simulink model "LED_TX"  (R2017b)
settings: Solver=VariableStepAuto  StartTime=0.0  StopTime=8099  RelTol=1e-3
undefined symbols (not defined in the file or in its folder): get, hot
libraries: visionsources x3, simulink x3, SimulinkLED1v4 x3, dspsnks4 x1
settings Model: Creator=asus  LastModifiedBy=asus

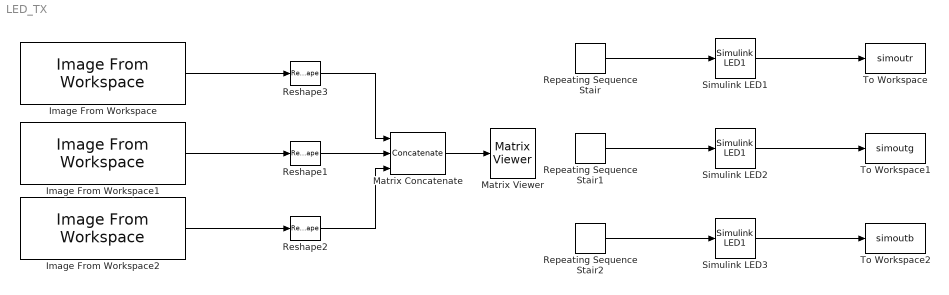
== system LED_TX ==
  Image From Workspace : visionsources/Image From Workspace  Tag=vipblks_nd  ImageValue=simoutr  Ts=1  imagePorts=One multidimensional signal  OutPortLabels=R  ImageDataType=Inherit from 'Value'  Signed=on  WordLength=16  sdImageDataType=sfix(16)  FractionLengthMode=User-defined  FractionLength=15
      settings: SourceProductName=Computer Vision System Toolbox  SourceProductBaseCode=VP
  Image From Workspace1 : visionsources/Image From Workspace  Tag=vipblks_nd  ImageValue=simoutg  Ts=1  imagePorts=One multidimensional signal  OutPortLabels=G  ImageDataType=Inherit from 'Value'  Signed=on  WordLength=16  sdImageDataType=sfix(16)  FractionLengthMode=User-defined  FractionLength=15
      settings: SourceProductName=Computer Vision System Toolbox  SourceProductBaseCode=VP
  Image From Workspace2 : visionsources/Image From Workspace  Tag=vipblks_nd  ImageValue=simoutb  Ts=1  imagePorts=One multidimensional signal  OutPortLabels=B  ImageDataType=Inherit from 'Value'  Signed=on  WordLength=16  sdImageDataType=sfix(16)  FractionLengthMode=User-defined  FractionLength=15
      settings: SourceProductName=Computer Vision System Toolbox  SourceProductBaseCode=VP
  Matrix Concatenate : Concatenate  NumInputs=3  Mode=Multidimensional array  ConcatenateDimension=2
  Matrix Viewer : dspsnks4/Matrix Viewer  ImageParams=off  CMapStr=hot(256)  AxisColorbar=off  AxisParams=off  AxisOrigin=Upper left corner  AxisTickMode=Auto  XTickRange=[0 1]  YTickRange=[0 1]  XLabel=RGB colors  YLabel=Pixel values  ZLabel=Z-axis  FigPos=get(0,'defaultfigureposition')  AxisZoom=off
      settings: SourceProductName=DSP System Toolbox  SourceProductBaseCode=DS  YMin=0  YMax=255
  Repeating Sequence Stair : simulink/Sources/Repeating Sequence Stair  OutValues=[251,107,54,59,59,59,59,59,59,59,59,59,59,59,59,59,59,59,59,59,59,59,59,59,59,59,59,59,59,59,59,59,59,59,59,59,59,59,59,59,59,59,54,107,255,198,56,59,59,59,59,59,59,59,59,59,59,59,59,59,59,59,59,59,59,59,59,59,59,59,59,59,59,59,59,59,59,59,59,59,59,59,59,59,59,59,59,59,56,204,156,51,59,59,59,59,59,59,59,59,59,59,59,59,59,59,59,59,59,59,59,58,58,58,58,59,59,59,59,59,59,59,59,59,59,59,59,59,59,59,59,59,59,51,154,125,53,59,59,59,59,59,59,59,59,59,59,59,59,59,59,59,59,59,58,58,58,58,58,58,58,58,59,59,59,59,59,59,59,59,59,59,59,59,59,59,59,59,54,113,99,55,59,59,59,59,59,59,59,59,59,59,59,59,59,59,59,59,58,58,58,58,58,58,58,58,58,58,59,59,59,59,59,59,59,59,59,59,59,59,59,59,59,56,85,82,57,59,59,59,59,59,59,59,59,59,59,59,59,59,59,59,58,58,58,58,58,58,58,58,58,58,58,58,59,59,59,59,59,59,59,59,59,59,59,59,59,59,58,70,69,58,59,59,59,59,59,59,59,59,59,59,59,59,59,59,58,58,58,58,58,58,57,57,58,58,58,58,58,58,59,59,59,59,59,59,59,59,59,59,59,59,59,59,60,60,59,59,59,59,59,59,59,59,59,59,59,59,59,59,59,58,58,58,58,57,57,57,57,57,57,58,58,58,58,58,59,59,59,59,59,59,59,59,59,59,59,59,59,59,59,59,59,59,59,59,59,59,59,59,59,59,59,59,59,58,58,58,58,57,57,57,57,57,57,57,57,57,58,58,58,59,59,59,59,59,59,59,59,59,59,59,59,59,59,59,59,59,59,59,59,59,59,59,59,59,59,59,59,58,58,58,58,57,57,57,57,57,57,57,57,57,57,57,58,58,58,59,59,59,59,59,59,59,59,59,59,59,59,59,59,59,59,59,59,59,59,59,59,59,59,59,59,59,58,58,58,57,57,57,56,56,56,56,56,56,57,57,57,57,58,58,58,59,59,59,59,59,59,59,59,59,59,59,59,59,59,59,59,59,59,59,59,59,59,59,59,59,58,58,58,57,57,57,56,56,56,56,56,56,56,56,56,57,57,58,58,58,59,59,59,59,59,59,59,59,59,59,59,59,59,59,59,59,59,59,59,59,59,59,59,59,59,58,58,58,57,57,56,56,56,56,56,56,56,56,56,56,56,57,57,58,58,58,59,59,59,59,59,59,59,59,59,59,59,59,59,59,59,59,59,59,59,59,59,59,59,58,58,58,57,57,56,56,56,55,55,55,55,55,55,56,56,56,57,57,57,58,58,59,59,59,59,59,59,59,59,59,59,59,59,59,59,59,59,59,59,59,59,59,59,59,58,58,57,57,56,56,56,55,55,55,55,55,55,55,55,56,56,56,57,57,58,58,58,59,59,59,59,59,59,59,59,59,59,59,59,59,59,59,59,59,59,59,59,59,59,58,58,57,56,56,56,55,55,55,54,54,54,54,54,55,55,56,56,56,57,57,58,58,59,59,59,59,59,59,59,59,59,59,59,59,59,59,59,59,59,59,59,59,59,58,58,57,57,56,56,55,55,54,54,54,54,54,54,54,54,55,55,56,56,56,57,58,58,59,59,59,59,59,59,59,59,59,59,59,59,59,59,59,59,59,59,59,59,59,58,58,57,56,56,55,55,54,54,54,54,53,53,53,54,54,54,55,55,56,56,57,57,58,58,59,59,59,59,59,59,59,59,59,59,59,59,59,59,59,59,59,59,59,58,58,57,57,56,56,55,54,54,54,53,53,53,53,53,53,53,54,54,55,55,56,56,57,58,58,59,59,59,59,59,59,59,59,59,59,59,59,59,59,59,59,59,59,59,58,58,57,56,56,55,55,54,54,52,60,103,122,104,60,52,53,53,54,54,55,56,56,57,58,58,59,59,59,59,59,59,59,59,59,59,59,59,59,59,59,59,59,59,59,58,58,57,56,56,55,54,53,52,121,208,221,219,220,209,122,53,53,53,54,54,55,56,57,57,58,58,59,59,59,59,59,59,59,59,59,59,59,59,59,59,59,59,59,58,58,57,57,56,55,54,53,55,154,222,219,219,220,220,220,224,156,55,52,53,54,55,56,56,57,58,58,59,59,59,59,59,59,59,59,59,59,59,59,59,59,59,59,59,58,58,57,56,56,55,54,51,150,223,219,219,220,220,220,220,220,225,151,51,53,54,54,55,56,56,57,58,59,59,59,59,59,59,59,59,59,59,59,59,59,59,59,59,59,58,58,57,56,55,54,49,118,221,219,220,220,220,221,221,221,221,221,222,119,48,53,54,55,56,56,57,58,58,59,59,59,59,59,59,59,59,59,59,59,59,59,59,59,58,58,57,56,56,55,51,76,205,221,219,220,220,221,221,221,221,221,221,223,208,77,50,54,54,55,56,57,58,58,59,59,59,59,59,59,59,59,59,59,59,59,59,59,59,58,58,57,56,55,54,51,161,224,219,220,221,221,222,222,222,222,222,222,221,226,163,51,53,54,55,56,57,57,58,59,59,59,59,59,59,59,59,59,59,59,59,59,59,59,58,58,56,56,55,50,95,217,220,220,220,221,222,222,222,223,223,222,222,222,222,220,96,48,54,54,56,56,57,58,58,59,59,59,59,59,59,59,59,59,59,59,59,59,59,58,57,56,56,54,52,169,224,219,220,221,222,222,223,223,223,223,223,223,222,222,226,172,52,53,54,55,56,57,58,58,59,59,59,59,59,59,59,59,59,59,59,59,59,58,58,57,56,55,50,92,217,220,220,221,222,222,223,223,223,224,224,224,223,223,223,223 ...(+23997 chars)]  tsamp=1  OutMin=[]  OutMax=[]  OutDataTypeStr=double  OutputDataTypeScalingMode=double  OutDataType=fixdt(0,8)  ConRadixGroup=Best Precision: Vector-wise  OutScaling=2^-12
  Repeating Sequence Stair1 : simulink/Sources/Repeating Sequence Stair  OutValues=[251,130,85,89,89,89,89,89,89,89,89,89,89,89,89,89,89,89,89,89,89,89,88,88,89,89,89,89,89,89,89,89,89,89,89,89,89,89,89,89,89,89,85,130,255,207,86,89,89,89,89,89,89,89,89,89,89,89,89,89,89,89,89,89,89,88,88,88,88,88,88,88,89,89,89,89,89,89,89,89,89,89,89,89,89,89,89,89,87,212,171,82,89,89,89,89,89,89,89,89,89,89,89,89,89,89,89,89,89,88,88,88,88,88,88,88,88,88,89,89,89,89,89,89,89,89,89,89,89,89,89,89,89,83,170,145,84,89,89,89,89,89,89,89,89,89,89,89,89,89,89,89,89,88,88,88,88,88,88,88,88,88,88,88,89,89,89,89,89,89,89,89,89,89,89,89,89,89,85,135,123,85,89,89,89,89,89,89,89,89,89,89,89,89,89,89,89,88,88,88,88,88,87,87,88,88,88,88,88,88,89,89,89,89,89,89,89,89,89,89,89,89,89,87,111,108,87,89,89,89,89,89,89,89,89,89,89,89,89,89,89,88,88,88,88,87,87,87,87,87,87,88,88,88,88,88,89,89,89,89,89,89,89,89,89,89,89,89,88,99,97,88,89,89,89,89,89,89,89,89,89,89,89,89,89,88,88,88,88,87,87,87,87,87,87,87,87,87,88,88,88,89,89,89,89,89,89,89,89,89,89,89,89,89,90,90,89,89,89,89,89,89,89,89,89,89,89,89,89,88,88,88,88,87,87,87,87,86,86,86,87,87,87,87,88,88,88,89,89,89,89,89,89,89,89,89,89,89,89,89,89,89,89,89,89,89,89,89,89,89,89,89,89,89,88,88,88,87,87,87,86,86,86,86,86,86,86,87,87,87,88,88,88,89,89,89,89,89,89,89,89,89,89,89,89,89,89,89,89,89,89,89,89,89,89,89,89,89,88,88,88,87,87,87,86,86,86,86,86,86,86,86,86,87,87,88,88,88,89,89,89,89,89,89,89,89,89,89,89,89,89,89,89,89,89,89,89,89,89,89,89,89,89,88,88,87,87,87,86,86,85,85,85,85,85,85,86,86,86,87,87,88,88,88,89,89,89,89,89,89,89,89,89,89,89,89,89,89,89,89,89,89,89,89,89,89,89,88,88,88,87,87,86,86,85,85,85,84,84,85,85,85,85,86,86,87,87,88,88,89,89,89,89,89,89,89,89,89,89,89,89,89,89,89,89,89,89,89,89,89,89,89,88,88,87,87,86,86,85,85,84,84,84,84,84,84,85,85,85,86,87,87,88,88,88,89,89,89,89,89,89,89,89,89,89,89,89,89,89,89,89,89,89,89,89,89,88,88,88,87,86,86,85,85,84,83,83,83,83,83,83,84,84,85,86,86,87,87,88,88,89,89,89,89,89,89,89,89,89,89,89,89,89,89,89,89,89,89,89,89,89,88,88,87,87,86,85,85,84,83,83,83,82,82,82,83,83,83,84,85,86,86,87,88,88,89,89,89,89,89,89,89,89,89,89,89,89,89,89,89,89,89,89,89,89,89,88,88,87,86,85,85,84,83,83,82,82,82,82,82,82,83,83,83,85,85,86,87,87,88,88,89,89,89,89,89,89,89,89,89,89,89,89,89,89,89,89,89,89,89,88,88,87,87,86,85,84,83,83,82,82,81,81,81,81,82,82,82,83,83,85,86,86,87,88,88,89,89,89,89,89,89,89,89,89,89,89,89,89,89,89,89,89,89,89,88,88,87,86,85,84,83,83,82,81,81,81,81,81,81,81,81,82,82,83,84,85,86,87,87,88,88,89,89,89,89,89,89,89,89,89,89,89,89,89,89,89,89,89,89,88,87,87,86,85,84,83,82,81,81,81,80,80,80,80,80,81,81,82,82,83,84,85,86,87,88,88,89,89,89,89,89,89,89,89,89,89,89,89,89,89,89,89,89,88,88,87,86,85,84,83,82,81,81,79,86,122,138,122,86,79,80,81,81,82,83,84,85,86,87,88,88,89,89,89,89,89,89,89,89,89,89,89,89,89,89,89,89,89,88,88,87,86,85,84,82,82,81,80,137,210,220,219,220,210,137,80,80,81,81,82,83,84,85,87,87,88,88,89,89,89,89,89,89,89,89,89,89,89,89,89,89,89,89,88,87,87,86,84,83,82,80,82,165,222,219,219,220,220,220,223,166,82,79,81,81,82,84,85,86,87,88,88,89,89,89,89,89,89,89,89,89,89,89,89,89,89,89,88,88,87,86,85,84,82,81,79,161,222,219,219,220,220,220,220,220,224,162,78,80,81,82,83,84,86,87,88,88,89,89,89,89,89,89,89,89,89,89,89,89,89,89,89,88,88,87,86,84,83,82,77,134,220,219,220,220,220,221,221,221,221,221,222,135,76,80,82,82,84,85,86,87,88,88,89,89,89,89,89,89,89,89,89,89,89,89,89,89,88,87,86,85,84,82,79,99,207,220,219,220,220,221,221,221,221,221,221,222,210,99,77,81,82,83,85,86,87,88,88,89,89,89,89,89,89,89,89,89,89,89,89,89,88,88,87,86,85,83,82,79,171,223,219,220,221,221,222,222,222,222,222,222,221,225,172,78,80,81,82,84,86,87,88,88,89,89,89,89,89,89,89,89,89,89,89,89,89,88,88,87,86,84,83,78,115,217,220,220,220,221,222,222,222,223,223,222,222,222,222,220,115,76,81,82,84,85,86,87,88,89,89,89,89,89,89,89,89,89,89,89,89,89,88,88,86,85,84,82,80,177,223,219,220,221,222,222,223,223,223,223,223,223,222,222,226,179,78,80,82,83,84,86,87,88,88,89,89,89,89,89,89,89,89,89,89,89,89,88,87,86,85,83,78,113,217,220,220,221,222,222,223,223,223,224,224,224,223,223 ...(+24118 chars)]  tsamp=1  OutMin=[]  OutMax=[]  OutDataTypeStr=double  OutputDataTypeScalingMode=double  OutDataType=fixdt(0,8)  ConRadixGroup=Best Precision: Vector-wise  OutScaling=2^-12
  Repeating Sequence Stair2 : simulink/Sources/Repeating Sequence Stair  OutValues=[253,177,150,152,152,152,152,152,152,152,152,152,152,152,152,152,152,152,151,151,151,151,151,151,151,151,151,151,151,152,152,152,152,152,152,152,152,152,152,152,152,152,150,177,255,225,150,152,152,152,152,152,152,152,152,152,152,152,152,152,152,152,151,151,151,151,151,151,151,151,151,151,151,151,151,152,152,152,152,152,152,152,152,152,152,152,152,152,150,228,203,148,152,152,152,152,152,152,152,152,152,152,152,152,152,152,151,151,151,151,151,150,150,150,150,151,151,151,151,151,151,152,152,152,152,152,152,152,152,152,152,152,152,148,202,187,149,152,152,152,152,152,152,152,152,152,152,152,152,152,151,151,151,151,150,150,150,150,150,150,150,150,151,151,151,151,152,152,152,152,152,152,152,152,152,152,152,152,149,180,173,150,152,152,152,152,152,152,152,152,152,152,152,152,151,151,151,151,150,150,150,150,149,149,150,150,150,150,151,151,151,151,152,152,152,152,152,152,152,152,152,152,152,151,166,164,151,152,152,152,152,152,152,152,152,152,152,152,152,151,151,151,150,150,150,149,149,148,148,149,149,150,150,150,151,151,151,151,152,152,152,152,152,152,152,152,152,152,151,158,157,151,152,152,152,152,152,152,152,152,152,152,152,151,151,151,150,150,150,149,148,148,148,148,148,148,148,149,150,150,151,151,151,152,152,152,152,152,152,152,152,152,152,152,153,152,152,152,152,152,152,152,152,152,152,152,152,152,151,151,151,150,150,149,148,148,148,147,147,147,148,148,148,149,150,150,151,151,151,152,152,152,152,152,152,152,152,152,152,152,152,152,152,152,152,152,152,152,152,152,152,152,151,151,151,150,150,149,148,148,147,147,147,147,147,147,147,148,148,149,150,151,151,151,152,152,152,152,152,152,152,152,152,152,152,152,152,152,152,152,152,152,152,152,152,152,152,151,151,150,150,149,148,147,147,147,146,146,146,146,146,147,147,148,148,150,150,151,151,151,152,152,152,152,152,152,152,152,152,152,152,152,152,152,152,152,152,152,152,152,152,151,151,151,150,149,148,147,147,146,145,145,145,145,145,145,145,147,147,148,148,150,150,151,151,152,152,152,152,152,152,152,152,152,152,152,152,152,152,152,152,152,152,152,152,152,151,151,150,150,148,148,147,146,145,145,144,144,144,144,144,145,145,146,147,148,149,150,151,151,151,152,152,152,152,152,152,152,152,152,152,152,152,152,152,152,152,152,152,152,151,151,151,150,149,148,147,146,145,144,144,143,143,143,143,143,144,145,145,147,148,148,150,150,151,151,152,152,152,152,152,152,152,152,152,152,152,152,152,152,152,152,152,152,152,151,151,150,149,148,147,146,145,144,143,143,143,142,142,142,143,143,144,144,146,147,148,149,150,151,151,151,152,152,152,152,152,152,152,152,152,152,152,152,152,152,152,152,152,152,151,151,150,149,148,147,145,144,143,143,141,141,141,141,141,141,142,143,144,145,146,147,148,149,150,151,151,152,152,152,152,152,152,152,152,152,152,152,152,152,152,152,152,152,151,151,151,150,148,147,146,144,144,142,141,141,140,140,140,140,140,141,142,143,144,145,146,148,149,150,151,151,152,152,152,152,152,152,152,152,152,152,152,152,152,152,152,152,152,151,151,150,149,148,146,145,144,142,141,140,140,139,139,139,139,139,140,141,142,143,144,146,147,148,150,151,151,151,152,152,152,152,152,152,152,152,152,152,152,152,152,152,152,152,151,151,150,148,147,145,144,143,141,140,139,138,138,138,138,138,138,139,140,141,142,144,144,146,148,149,150,151,151,152,152,152,152,152,152,152,152,152,152,152,152,152,152,152,151,151,150,149,148,146,144,143,142,141,139,138,138,137,137,137,137,137,138,139,140,141,142,144,145,147,148,150,151,151,152,152,152,152,152,152,152,152,152,152,152,152,152,152,152,151,151,150,149,147,145,144,142,141,139,138,137,141,161,170,161,140,136,137,138,139,140,141,143,144,146,148,149,151,151,151,152,152,152,152,152,152,152,152,152,152,152,152,152,152,151,151,149,148,146,145,143,141,140,138,137,170,213,220,219,220,214,170,136,137,138,139,140,142,144,145,147,149,150,151,151,152,152,152,152,152,152,152,152,152,152,152,152,152,151,151,150,149,148,146,144,142,140,138,138,187,220,219,219,220,220,220,222,187,137,137,138,139,141,143,145,147,148,150,151,151,152,152,152,152,152,152,152,152,152,152,152,152,152,151,151 ...(+28404 chars)]  tsamp=1  OutMin=[]  OutMax=[]  OutDataTypeStr=double  OutputDataTypeScalingMode=double  OutDataType=fixdt(0,8)  ConRadixGroup=Best Precision: Vector-wise  OutScaling=2^-12
  Reshape1 : Reshape  OutputDimensionality=Customize  OutputDimensions=[90,90]
  Reshape2 : Reshape  OutputDimensionality=Customize  OutputDimensions=[90,90]
  Reshape3 : Reshape  OutputDimensionality=Customize  OutputDimensions=[90,90]
  Simulink LED1 : SimulinkLED1v4/Simulink LED1  Description=|  outportflag=on  IconShape=Triangle  range1=[0 255]  color1=Red  range2=[100 255]  color2=Green  colorRest=Blue
      | -ranges-
      | (-inf 0]
      settings: AttributesFormatString=%<Description>  SourceProductName=The database C:\Users\asus\AppData\Roaming\MathWorks\MATLAB\R2017b\slblocks_master.db is locked, or a table in the database is locked. (database is locked)
  Simulink LED2 : SimulinkLED1v4/Simulink LED1  Description=|  outportflag=on  IconShape=Triangle  range1=[0 255]  color1=Red  range2=[100 255]  color2=Green  colorRest=Blue
      | -ranges-
      | (-inf 0]
      settings: AttributesFormatString=%<Description>  SourceProductName=The database C:\Users\asus\AppData\Roaming\MathWorks\MATLAB\R2017b\slblocks_master.db is locked, or a table in the database is locked. (database is locked)
  Simulink LED3 : SimulinkLED1v4/Simulink LED1  Description=|  outportflag=on  IconShape=Triangle  range1=[0 255]  color1=Red  range2=[100 255]  color2=Green  colorRest=Blue
      | -ranges-
      | (-inf 0]
      settings: AttributesFormatString=%<Description>  SourceProductName=The database C:\Users\asus\AppData\Roaming\MathWorks\MATLAB\R2017b\slblocks_master.db is locked, or a table in the database is locked. (database is locked)
  To Workspace : ToWorkspace  VariableName=simoutr  SampleTime=1
      settings: Save2DSignal=2-D array (concatenate along first dimension)
  To Workspace1 : ToWorkspace  VariableName=simoutg  SampleTime=1
      settings: Save2DSignal=2-D array (concatenate along first dimension)
  To Workspace2 : ToWorkspace  VariableName=simoutb  SampleTime=1
      settings: Save2DSignal=2-D array (concatenate along first dimension)
  wires:
  Repeating Sequence Stair1/1 -> Simulink LED2/1
  Simulink LED2/1 -> To Workspace1/1
  Repeating Sequence Stair/1 -> Simulink LED1/1
  Repeating Sequence Stair2/1 -> Simulink LED3/1
  Simulink LED1/1 -> To Workspace/1
  Simulink LED3/1 -> To Workspace2/1
  Reshape2/1 -> Matrix Concatenate/3
  Image From Workspace/1 -> Reshape3/1
  Reshape1/1 -> Matrix Concatenate/2
  Image From Workspace1/1 -> Reshape1/1
  Matrix Concatenate/1 -> Matrix Viewer/1
  Image From Workspace2/1 -> Reshape2/1
  Reshape3/1 -> Matrix Concatenate/1
